simulink model "CurveLowVel"  (R2024b)
settings: Solver=FixedStepAuto  StartTime=0.0  StopTime=Ts  FixedStep=0.001  RelTol=1e-3
PreLoadFcn:
  | setUpCurveLowVel
model workspace (MAT data in the model file):
  firstWarning = 0
  originalScenarioChecksum = 'F73A6DA3C723D3CA73A6F931B7A52A9C'
values from neighbouring files (symbols this model uses):
  K = lqr(A,B,Q,R)    [LQR_Coeff_Low_Vel.m]
  psi_o = 0    [setUpCurveLowVel.m]
  X_o = refPose(1,1)    [setUpCurveLowVel.m]
  xRef = refPose(:,1)    [setUpCurveLowVel.m]
  Y_o = -refPose(1,2)    [setUpCurveLowVel.m]
  yRef = -refPose(:,2)    [setUpCurveLowVel.m]
libraries: simulink x6, slpidlib x2, vehdynlibviscommon x1, autolibshared x1
settings Model: PacingRate=0.700000  Creator=valakshe  LastModifiedBy=Karthik R
settings SolverCC: AlgebraicLoopSolver=TrustRegion
settings OptimizationCC: OptimizeBlockIOStorage=off  OptimizeDataStoreBuffers=off  BusAssignmentInplaceUpdate=off
settings DebuggingCC: UnconnectedInputMsg=warning  UnconnectedOutputMsg=warning  UnconnectedLineMsg=warning  SFUnexpectedBacktrackingDiag=warning  SFNoUnconditionalDefaultTransitionDiag=warning
settings ModelReferenceCC: EnableRefExpFcnMdlSchedulingChecks=on
settings RTWCC: GenerateReport=on  BuildConfiguration=Debug  LaunchReport=on  GPUComputeCapability=3.5  DLArmComputeVersion=19.05
settings CodeAppCC: ForceParamTrailComments=on  MATLABSourceComments=on  EnableCustomComments=on
settings GRTTargetCC: CombineSignalStateStructs=on  SupportVariableSizeSignals=on  MultiInstanceErrorCode=Warning

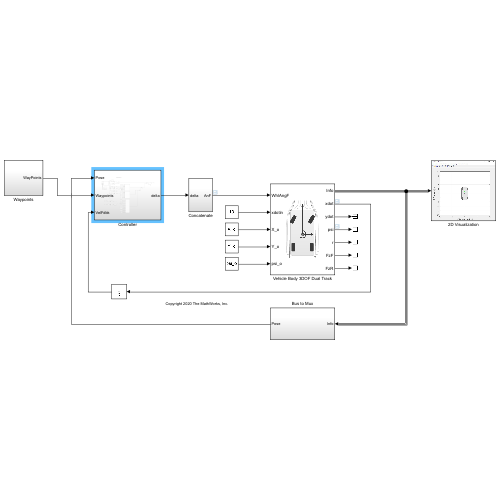
[thumbnail: Simulink's stored preview of the top-level diagram]
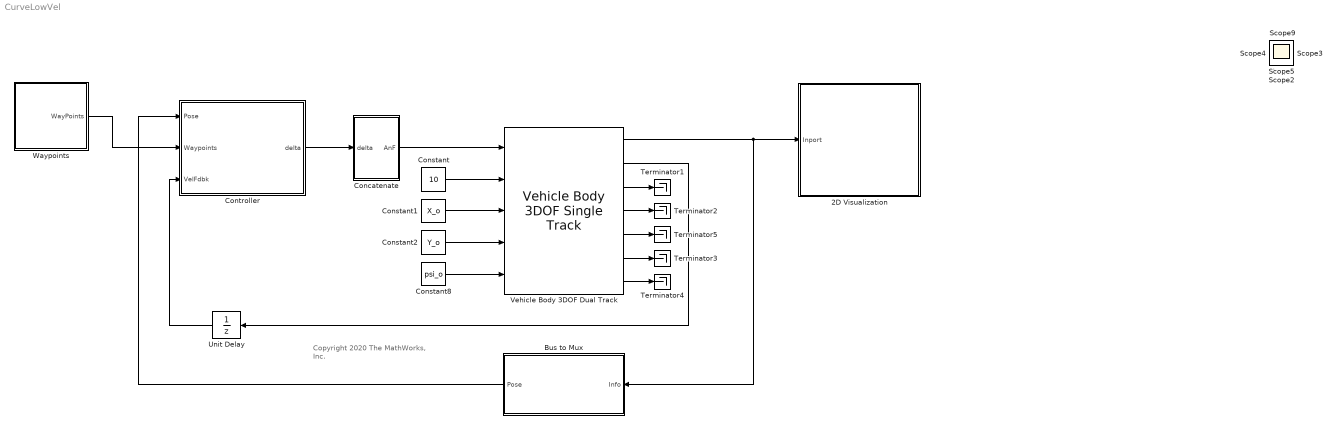
== system CurveLowVel ==
  note: Copyright 2020 The MathWorks, Inc.
  2D Visualization : Subsystem
      mask Display: image("visualization.JPG");
  Bus to Mux : Subsystem
  Concatenate : Subsystem
  Constant : Constant  Value=10
  Constant1 : Constant  Value=X_o
  Constant2 : Constant  Value=Y_o
  Constant8 : Constant  Value=psi_o
  Controller : Subsystem
  Terminator{1..5} (5 alike) : Terminator
  Unit Delay : UnitDelay  SampleTime=-1  HasFrameUpgradeWarning=on
  Vehicle Body 3DOF Dual Track : autolibshared/Vehicle Body 3DOF Single Track  trackMode=Dual  inputMode=External longitudinal velocity  frontSteerMode=on  rearSteerMode=off  windMode=off  muMode=off  extFMode=off  extMMode=off  htchFMode=off  htchMMode=off  extXo=on  extpsio=on  extxdoto=off  extro=off  extYo=on  extTamb=off  extydoto=off  aMode=2  NF=2  NR=2  m=2000  a=1.4  b=1.6  h=0.35  dh=1  hh=0.2  X_o=0  xdot_o=0  CalphaMode=off  sigmaMode=on  d=0  hl=0  w=[1.4,1.4]  Cy_f=12e3  Cy_r=11e3  sigma_f=.1  sigma_r=.1  alpha_f_brk=[-.1 .1]  Cy_f_data=[-9e3 9e3]  alpha_r_brk=[-.1 .1]  Cy_r_data=[-9e3 9e3]  Y_o=0  ydot_o=0  Izz=4000  psi_o=0  r_o=0  Af=2  Cd=.3  Cl=.1  Cpm=.1  beta_w=[0:0.01:0.3]  Cs=[0:0.03:0.9]  Cym=[0:0.01:0.3]  Pabs=101325  Tair=273  g=9.81  mu=1  xdot_tol=.01  Fznom=5000  Fxtire_sat=7e4  Fytire_sat=7e4  longOff=0  latOff=0  vertOff=0  wrapAng=off
  Waypoints : Subsystem
  Scope{,1..5,9} (7 alike) : Scope
  wires:
  Vehicle Body 3DOF Dual Track/7 -> Terminator4/1
  Vehicle Body 3DOF Dual Track/3 -> Terminator1/1
  Constant1/1 -> Vehicle Body 3DOF Dual Track/3
  Vehicle Body 3DOF Dual Track/6 -> Terminator3/1
  Constant2/1 -> Vehicle Body 3DOF Dual Track/4
  Concatenate/1(AnF) -> Vehicle Body 3DOF Dual Track/1
  Constant8/1 -> Vehicle Body 3DOF Dual Track/5
  Vehicle Body 3DOF Dual Track/1 -> 2D Visualization/1(Inport), Bus to Mux/1(Info)
  Controller/1(delta) -> Concatenate/1(delta)
  Bus to Mux/1(Pose) -> Controller/1(Pose)
  Constant/1 -> Vehicle Body 3DOF Dual Track/2
  Vehicle Body 3DOF Dual Track/4 -> Terminator2/1
  Vehicle Body 3DOF Dual Track/5 -> Terminator5/1
  Vehicle Body 3DOF Dual Track/2 -> Unit Delay/1
  Waypoints/1(WayPoints) -> Controller/2(Waypoints)
  Unit Delay/1 -> Controller/3(VelFdbk)

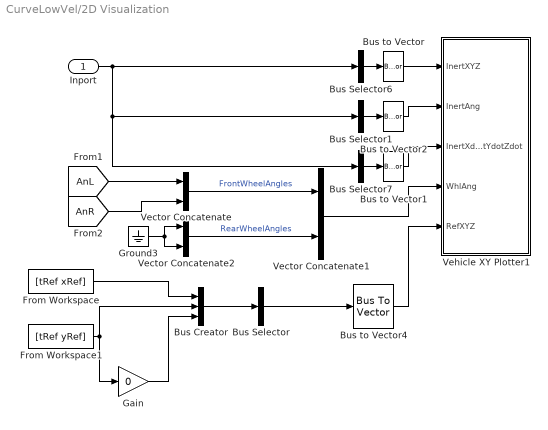
== system CurveLowVel/2D Visualization ==
  Inport : Inport
  Bus Creator : BusCreator  Inputs=3
  Bus Selector : BusSelector  OutputSignals=signal1,signal2,signal3  OutputAsBus=on
  Bus Selector1 : BusSelector  OutputSignals=InertFrm.Cg.Ang.phi,InertFrm.Cg.Ang.theta,InertFrm.Cg.Ang.psi  OutputAsBus=on
  Bus Selector6 : BusSelector  OutputSignals=InertFrm.Geom.Disp.X,InertFrm.Geom.Disp.Y,InertFrm.Geom.Disp.Z  OutputAsBus=on
  Bus Selector7 : BusSelector  OutputSignals=InertFrm.Geom.Vel.Xdot,InertFrm.Geom.Vel.Ydot,InertFrm.Geom.Vel.Zdot  OutputAsBus=on
  Bus to Vector{,1..2,4} (4 alike) : BusToVector
  From Workspace : FromWorkspace  VariableName=[tRef xRef]
  From Workspace1 : FromWorkspace  VariableName=[tRef yRef]
  Gain : Gain  Gain=0
  Ground3 : Ground
  Vector Concatenate : Concatenate
  Vector Concatenate1 : Concatenate
  Vector Concatenate2 : Concatenate
  Vehicle XY Plotter1 : Subsystem  mask(Vehicle XY Plotter){extRef=on, extStats=off, extTireF=off, a=2, b=2, w=2, figBorder=10, bufferSize=1024, velNorm=5, tireFNorm=1000, pltDT=0.2}
      mask prompts: extRef "Plot path reference, extRef"; extStats "Display speed, RPM and Gear"; extTireF "Display tire forces"; a "Distance to front axle from CG, a [m]:"; b "Distance to rear axle from CG, b [m]:"; w "Track width, w [m]:"; figBorder "Distance to figure borders, figBorder [m]:"; bufferSize "Path buffer sampe size, bufferSize []:"; velNorm "Velocity vector scaling, velNorm [m*s/m]:"; tireFNorm "Tire force vector scaling, tireFNorm [m/N]:"; pltDT "Plot update rate, pltDT [s]:"
      mask help:
      | This block will display a MATLAB figure which indicates the vehicle path, current position and heading velocity.
      | An optional path reference is also provided.
      mask init:
      | block = gcb;
      | if autoblkschecksimstopped(block)
      |     ParamNames = {'extRef';'extStats';'extTireF';'extTireF'};
      |     PortNames = {'RefXYZ';'Stats';'TireFx';'TireFy'};
      |     for idx=1:length(PortNames)
      |         InportOption  = {'built-in/Ground', [PortNames{idx}, ' Ground'];...
      |             'built-in/Inport',PortNames{idx}};
      |         if ~strcmp(get_param(block,ParamNames{idx}),'on')
      |             NewBlkHdl = autoblksreplaceblock(block, InportOption, 1);
      |             set_param(NewBlkHdl, 'ShowName', 'off');
      |         else
      |             autoblksreplaceblock(block, InportOption, 2);
      |         end
      |     end
      |     InportNames = {'InertXYZ';'InertAng';'InertXdotYdotZdot';'WhlAng';'RefXYZ';'Stats';'TireFx';'TireFy'};
      |     FoundNames = get_param(find_system(block, 'LookUnderMasks', 'all', 'SearchDepth', 1, 'FollowLinks', 'on', 'BlockType', 'Inport'), 'Name');
      |     [~,PortI] = intersect(InportNames, FoundNames);
      |     PortI = sort(PortI);
      |     for idx = 1:length(PortI)
      |         set_param([block, '/', InportNames{PortI(idx)}], 'Port', num2str(idx));
      |     end
      | end
      mask TypeOptions a: Vehicle XY Plotter/a
      mask TypeOptions b: Vehicle XY Plotter/b
      mask TypeOptions w: Vehicle XY Plotter/w
      mask TypeOptions figBorder: Vehicle XY Plotter/figBorder
      mask TypeOptions bufferSize: Vehicle XY Plotter/bufferSize
      mask TypeOptions velNorm: Vehicle XY Plotter/velNorm
      mask TypeOptions tireFNorm: Vehicle XY Plotter/tireFNorm
      mask DialogControl Container3 Prompt: Plot and Display Options
  wires:
  Vector Concatenate1/1 -> Vehicle XY Plotter1/4(WhlAng)
  Ground3/1 -> Vector Concatenate2/1, Vector Concatenate2/2
  Bus Selector6/1 -> Bus to Vector/1
  Vector Concatenate/1 -> Vector Concatenate1/1  "FrontWheelAngles"
  [AnL] -> Vector Concatenate/1
  Vector Concatenate2/1 -> Vector Concatenate1/2  "RearWheelAngles"
  Bus Selector7/1 -> Bus to Vector1/1
  Bus to Vector1/1 -> Vehicle XY Plotter1/3(InertXdotYdotZdot)
  Bus to Vector/1 -> Vehicle XY Plotter1/1(InertXYZ)
  Bus to Vector2/1 -> Vehicle XY Plotter1/2(InertAng)
  Bus Selector1/1 -> Bus to Vector2/1
  [AnR] -> Vector Concatenate/2
  Inport/1 -> Bus Selector7/1, Bus Selector1/1, Bus Selector6/1
  Bus to Vector4/1 -> Vehicle XY Plotter1/5(RefXYZ)
  Bus Selector/1 -> Bus to Vector4/1
  From Workspace1/1 -> Gain/1, Bus Creator/2
  Gain/1 -> Bus Creator/3
  From Workspace/1 -> Bus Creator/1
  Bus Creator/1 -> Bus Selector/1

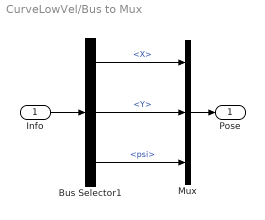
== system CurveLowVel/Bus to Mux ==
  Info : Inport
  Bus Selector1 : BusSelector  OutputSignals=InertFrm.Cg.Disp.X,InertFrm.Cg.Disp.Y,InertFrm.Cg.Ang.psi
  Mux : Mux  Inputs=3
  Pose : Outport
  wires:
  Bus Selector1/3 -> Mux/3  "<psi>"
  Bus Selector1/1 -> Mux/1  "<X>"
  Mux/1 -> Pose/1
  Bus Selector1/2 -> Mux/2  "<Y>"
  Info/1 -> Bus Selector1/1

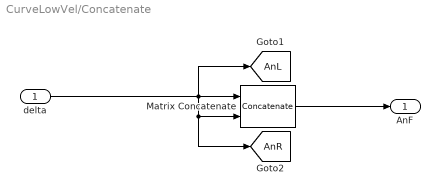
== system CurveLowVel/Concatenate ==
  delta : Inport
  Matrix Concatenate : Concatenate
  AnF : Outport  VectorParamsAs1DForOutWhenUnconnected=off
  tag scope: AnL=global, AnR=global
  wires:
  Matrix Concatenate/1 -> AnF/1
  delta/1 -> [AnL], [AnR], Matrix Concatenate/2, Matrix Concatenate/1

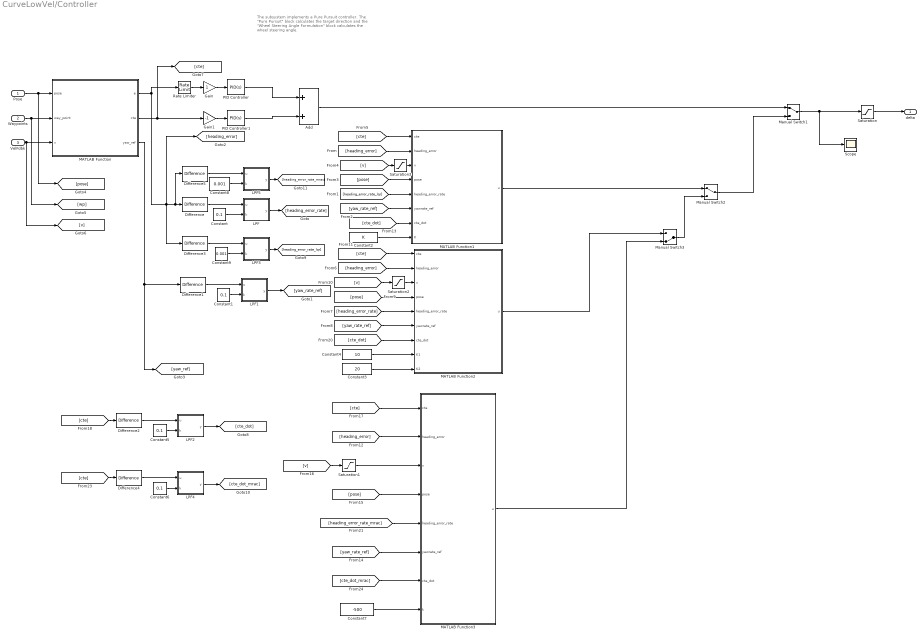
== system CurveLowVel/Controller ==
  note: The subsystem implements a Pure Pursuit controller. The "Pure Pursuit" block calculates the target direction and the "Wheel Steering Angle Formulation" block calculates the wheel steering angle.
  Pose : Inport
  Waypoints : Inport  Port=2
  VelFdbk : Inport  Port=3
  Add : Sum
  Constant{,1,5..6} (4 alike) : Constant  Value=0.1
  Constant2 : Constant  Value=K
  Constant3 : Constant  Value=20
  Constant4 : Constant  Value=10
  Constant7 : Constant  Value=-500
  Constant8 : Constant  Value=0.001
  Constant9 : Constant  Value=0.001
  Difference{,1..5} (6 alike) : simulink/Discrete/Difference  ICPrevInput=0.0  OutMin=[]  OutMax=[]  OutDataType=fixdt(1, 16)  OutScaling=2^-10  DoSatur=off
  Gain : Gain
  Gain1 : Gain  Gain=-1
  LPF : Subsystem
  LPF1 : Subsystem
  LPF2 : Subsystem
  LPF3 : Subsystem
  LPF4 : Subsystem
  LPF5 : Subsystem
  MATLAB Function : MATLAB Function  TreatAsAtomicUnit=on
  MATLAB Function1 : MATLAB Function  TreatAsAtomicUnit=on
  MATLAB Function2 : MATLAB Function  TreatAsAtomicUnit=on
  MATLAB Function3 : MATLAB Function  TreatAsAtomicUnit=on
  Manual Switch1 : ManualSwitch
  Manual Switch2 : ManualSwitch
  Manual Switch3 : ManualSwitch  CurrentSetting=0
  PID Controller : slpidlib/PID Controller  Controller=PID  Form=Parallel  TimeDomain=Continuous-time  UseExternalTs=off  SampleTime=-1  IntegratorMethod=Forward Euler  FilterMethod=Forward Euler  ControllerParametersSource=internal  P=0.7  I=0.002  UseKiTs=off  D=0  UseExternalDerivativeSource=off  N=100  UseFilter=on  TunerSelectOption=Transfer Function Based (PID Tuner App)  InitialConditionSource=internal  InitialConditionForIntegrator=0  InitialConditionForFilter=0  DifferentiatorICPrevScaledInput=0  ExternalReset=none  TrackingMode=off  Kt=1  LimitOutput=off  SatLimitsSource=internal  UpperSaturationLimit=inf  LowerSaturationLimit=-inf  LinearizeAsGain=on  AntiWindupMode=none  Kb=1  LimitIntegrator=off  UpperIntegratorSaturationLimit=inf  LowerIntegratorSaturationLimit=-inf  POutMin=[]  POutMax=[]  IOutMin=[]  IOutMax=[]  DOutMin=[]  DOutMax=[]  NOutMin=[]  NOutMax=[]  SumOutMin=[]  SumOutMax=[]  SaturationOutMin=[]  SaturationOutMax=[]  PParamMin=[]  PParamMax=[]  IParamMin=[]  IParamMax=[]  DParamMin=[]  DParamMax=[]  NParamMin=[]  NParamMax=[]  KbParamMin=[]  KbParamMax=[]  KtParamMin=[]  KtParamMax=[]  KbOutMin=[]  KbOutMax=[]  KtOutMin=[]  KtOutMax=[]  IntegratorOutMin=[]  IntegratorOutMax=[]  FilterOutMin=[]  FilterOutMax=[]  SumI1OutMin=[]  SumI1OutMax=[]  SumI2OutMin=[]  SumI2OutMax=[]  SumI3OutMin=[]  SumI3OutMax=[]  SumI4OutMin=[]  SumI4OutMax=[]  SumDOutMin=[]  SumDOutMax=[]  DifferentiatorOutMin=[]  DifferentiatorOutMax=[]  FilterDiffOutCoefMin=[]  FilterDiffOutCoefMax=[]  ReciprocalOutMin=[]  ReciprocalOutMax=[]  SumDenOutMin=[]  SumDenOutMax=[]  SumNumOutMin=[]  SumNumOutMax=[]  DivideOutMin=[]  DivideOutMax=[]  UdiffTsProdOutMin=[]  UdiffTsProdOutMax=[]  NTsProdOutMin=[]  NTsProdOutMax=[]  UintegralTsProdOutMin=[]  UintegralTsProdOutMax=[]  UngainTsProdOutMin=[]  UngainTsProdOutMax=[]  ClampingZeroOutDataTypeStr=Inherit: Inherit via back propagation  ClampingZeroOutMin=[]  ClampingZeroOutMax=[]  FilterDenConstantOutDataTypeStr=Inherit: Inherit via back propagation  FilterDenConstantOutMin=[]  FilterDenConstantOutMax=[]  PCopyOutDataTypeStr=Inherit: Inherit via back propagation  PCopyOutMin=[]  PCopyOutMax=[]  NCopyOutDataTypeStr=Inherit: Inherit via back propagation  NCopyOutMin=[]  NCopyOutMax=[]  IntegratorContinuousStateAttributes=''  IntegratorStateMustResolveToSignalObject=off  IntegratorRTWStateStorageClass=Auto  FilterContinuousStateAttributes=''  FilterStateMustResolveToSignalObject=off  FilterRTWStateStorageClass=Auto  ParallelPVariant=InternalParameters  IdealPVariant=Disabled  IVariant=InternalParameters  DVariant=InternalParameters  IntegratorVariant=Continuous  SatVariant=Disabled  AWVariant=Passthrough  PCopyVariant=Disabled  TRVariant=Disabled  FdbkBlocksVariant=Forward  IdealPFdbkVariant=Disabled  SatFdbkVariant=Disabled  DerivativeFilterVariant=ContFilter  NVariant=InternalParameters  NCopyVariant=Disabled  FilterICVariant=InternalICsFilter  IntegratorICVariant=InternalICs  ExternalResetVariant=Disabled  TRSumVariant=Passthrough  SumFdbkVariant=Disabled  SumVariant=Sum_PID  TsampFilterVariant=InternalTs  TsampNgainVariant=Passthrough  TsampIntegralVariant=Disabled_SignalSpec  ExternalSaturationOutDataTypeStr=Inherit: Same as second input  DerivativeSourceVariant=ErrorSignal  PreIntVariant=InternalPreInt
  PID Controller1 : slpidlib/PID Controller  Controller=PID  Form=Parallel  TimeDomain=Continuous-time  UseExternalTs=off  SampleTime=-1  IntegratorMethod=Forward Euler  FilterMethod=Forward Euler  ControllerParametersSource=internal  P=0.07  I=0.0002  UseKiTs=off  D=0  UseExternalDerivativeSource=off  N=100  UseFilter=on  TunerSelectOption=Transfer Function Based (PID Tuner App)  InitialConditionSource=internal  InitialConditionForIntegrator=0  InitialConditionForFilter=0  DifferentiatorICPrevScaledInput=0  ExternalReset=none  TrackingMode=off  Kt=1  LimitOutput=off  SatLimitsSource=internal  UpperSaturationLimit=inf  LowerSaturationLimit=-inf  LinearizeAsGain=on  AntiWindupMode=none  Kb=1  LimitIntegrator=off  UpperIntegratorSaturationLimit=inf  LowerIntegratorSaturationLimit=-inf  POutMin=[]  POutMax=[]  IOutMin=[]  IOutMax=[]  DOutMin=[]  DOutMax=[]  NOutMin=[]  NOutMax=[]  SumOutMin=[]  SumOutMax=[]  SaturationOutMin=[]  SaturationOutMax=[]  PParamMin=[]  PParamMax=[]  IParamMin=[]  IParamMax=[]  DParamMin=[]  DParamMax=[]  NParamMin=[]  NParamMax=[]  KbParamMin=[]  KbParamMax=[]  KtParamMin=[]  KtParamMax=[]  KbOutMin=[]  KbOutMax=[]  KtOutMin=[]  KtOutMax=[]  IntegratorOutMin=[]  IntegratorOutMax=[]  FilterOutMin=[]  FilterOutMax=[]  SumI1OutMin=[]  SumI1OutMax=[]  SumI2OutMin=[]  SumI2OutMax=[]  SumI3OutMin=[]  SumI3OutMax=[]  SumI4OutMin=[]  SumI4OutMax=[]  SumDOutMin=[]  SumDOutMax=[]  DifferentiatorOutMin=[]  DifferentiatorOutMax=[]  FilterDiffOutCoefMin=[]  FilterDiffOutCoefMax=[]  ReciprocalOutMin=[]  ReciprocalOutMax=[]  SumDenOutMin=[]  SumDenOutMax=[]  SumNumOutMin=[]  SumNumOutMax=[]  DivideOutMin=[]  DivideOutMax=[]  UdiffTsProdOutMin=[]  UdiffTsProdOutMax=[]  NTsProdOutMin=[]  NTsProdOutMax=[]  UintegralTsProdOutMin=[]  UintegralTsProdOutMax=[]  UngainTsProdOutMin=[]  UngainTsProdOutMax=[]  ClampingZeroOutDataTypeStr=Inherit: Inherit via back propagation  ClampingZeroOutMin=[]  ClampingZeroOutMax=[]  FilterDenConstantOutDataTypeStr=Inherit: Inherit via back propagation  FilterDenConstantOutMin=[]  FilterDenConstantOutMax=[]  PCopyOutDataTypeStr=Inherit: Inherit via back propagation  PCopyOutMin=[]  PCopyOutMax=[]  NCopyOutDataTypeStr=Inherit: Inherit via back propagation  NCopyOutMin=[]  NCopyOutMax=[]  IntegratorContinuousStateAttributes=''  IntegratorStateMustResolveToSignalObject=off  IntegratorRTWStateStorageClass=Auto  FilterContinuousStateAttributes=''  FilterStateMustResolveToSignalObject=off  FilterRTWStateStorageClass=Auto  ParallelPVariant=InternalParameters  IdealPVariant=Disabled  IVariant=InternalParameters  DVariant=InternalParameters  IntegratorVariant=Continuous  SatVariant=Disabled  AWVariant=Passthrough  PCopyVariant=Disabled  TRVariant=Disabled  FdbkBlocksVariant=Forward  IdealPFdbkVariant=Disabled  SatFdbkVariant=Disabled  DerivativeFilterVariant=ContFilter  NVariant=InternalParameters  NCopyVariant=Disabled  FilterICVariant=InternalICsFilter  IntegratorICVariant=InternalICs  ExternalResetVariant=Disabled  TRSumVariant=Passthrough  SumFdbkVariant=Disabled  SumVariant=Sum_PID  TsampFilterVariant=InternalTs  TsampNgainVariant=Passthrough  TsampIntegralVariant=Disabled_SignalSpec  ExternalSaturationOutDataTypeStr=Inherit: Same as second input  DerivativeSourceVariant=ErrorSignal  PreIntVariant=InternalPreInt
  Rate Limiter : RateLimiter  RisingSlewLimit=10  FallingSlewLimit=-10  SampleTimeMode=inherited
  Saturation : Saturate  UpperLimit=3  LowerLimit=-3
  Saturation1 : Saturate  UpperLimit=200  LowerLimit=1
  Saturation2 : Saturate  UpperLimit=200  LowerLimit=1
  Saturation3 : Saturate  UpperLimit=200  LowerLimit=3
  Scope : Scope
  delta : Outport
  wires:
  Waypoints/1 -> [wp], MATLAB Function/2(way_point)
  Pose/1 -> [pose], MATLAB Function/1(pose)
  Manual Switch1/1 -> Scope/1, Saturation/1
  VelFdbk/1 -> [v], MATLAB Function/3(v)
  Rate Limiter/1 -> Gain/1
  Gain/1 -> PID Controller/1
  Add/1 -> Manual Switch1/1
  PID Controller/1 -> Add/1
  PID Controller1/1 -> Add/2
  MATLAB Function/2(cte) -> [cte], Gain1/1
  Gain1/1 -> PID Controller1/1
  Difference/1 -> LPF/1(u)
  MATLAB Function/3(yaw_ref) -> [yaw_ref], Difference1/1
  Difference1/1 -> LPF1/1(u)
  Constant/1 -> LPF/2(k)
  Constant1/1 -> LPF1/2(k)
  Constant2/1 -> MATLAB Function1/8(K)
  MATLAB Function1/1(u) -> Manual Switch2/1
  Manual Switch2/1 -> Manual Switch1/2
  MATLAB Function2/1(u) -> Manual Switch3/1
  Constant3/1 -> MATLAB Function2/9(K2)
  Constant4/1 -> MATLAB Function2/8(K1)
  Saturation/1 -> delta/1
  MATLAB Function3/1(u) -> Manual Switch3/2
  Manual Switch3/1 -> Manual Switch2/2
  LPF/1(y) -> [heading_error_rate]
  LPF1/1(y) -> [yaw_rate_ref]
  [heading_error] -> MATLAB Function1/2(heading_error)
  [heading_error_rate_lqr] -> MATLAB Function1/5(heading_error_rate)
  [yaw_rate_ref] -> MATLAB Function1/6(yawrate_ref)
  [pose] -> MATLAB Function1/4(pose)
  [v] -> Saturation3/1
  [cte] -> MATLAB Function1/1(cte)
  [cte] -> MATLAB Function2/1(cte)
  [heading_error] -> MATLAB Function2/2(heading_error)
  [v] -> Saturation2/1
  [pose] -> MATLAB Function2/4(pose)
  [heading_error_rate] -> MATLAB Function2/5(heading_error_rate)
  [yaw_rate_ref] -> MATLAB Function2/6(yawrate_ref)
  [cte] -> MATLAB Function3/1(cte)
  [heading_error] -> MATLAB Function3/2(heading_error)
  [v] -> Saturation1/1
  [pose] -> MATLAB Function3/4(pose)
  [heading_error_rate_mrac] -> MATLAB Function3/5(heading_error_rate)
  [yaw_rate_ref] -> MATLAB Function3/6(yawrate_ref)
  LPF2/1(y) -> [cte_dot]
  [cte] -> Difference2/1
  Constant5/1 -> LPF2/2(k)
  Difference2/1 -> LPF2/1(u)
  [cte_dot_mrac] -> MATLAB Function3/7(cte_dot)
  Saturation1/1 -> MATLAB Function3/3(v)
  Saturation2/1 -> MATLAB Function2/3(v)
  Saturation3/1 -> MATLAB Function1/3(v)
  [cte_dot] -> MATLAB Function2/7(cte_dot)
  Constant7/1 -> MATLAB Function3/8(k)
  LPF3/1(y) -> [heading_error_rate_lqr]
  Difference3/1 -> LPF3/1(u)
  Constant9/1 -> LPF3/2(k)
  [cte_dot] -> MATLAB Function1/7(cte_dot)
  Difference4/1 -> LPF4/1(u)
  [cte] -> Difference4/1
  Constant6/1 -> LPF4/2(k)
  LPF4/1(y) -> [cte_dot_mrac]
  MATLAB Function/1(e) -> Difference3/1, [heading_error], Difference5/1, Difference/1, Rate Limiter/1
  LPF5/1(y) -> [heading_error_rate_mrac]
  Constant8/1 -> LPF5/2(k)
  Difference5/1 -> LPF5/1(u)

== system CurveLowVel/Waypoints ==
  Constant3 : Constant  Value=xRef  SampleTime=0.1
  Constant4 : Constant  Value=yRef  SampleTime=0.1
  Matrix Concatenate : Concatenate  Mode=Multidimensional array  ConcatenateDimension=2
  WayPoints : Outport
  wires:
  Constant4/1 -> Matrix Concatenate/2
  Constant3/1 -> Matrix Concatenate/1
  Matrix Concatenate/1 -> WayPoints/1

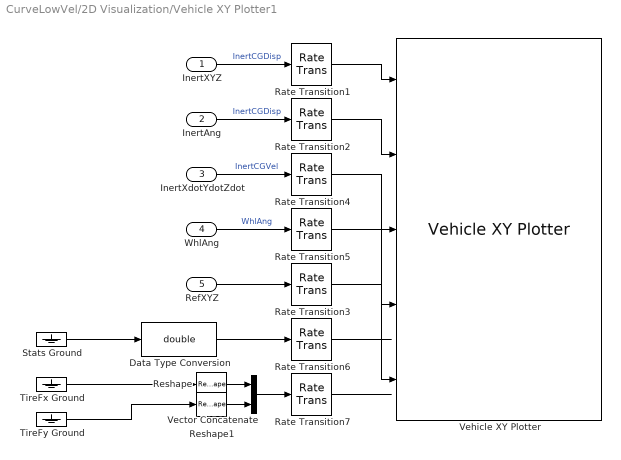
== system CurveLowVel/2D Visualization/Vehicle XY Plotter1 ==
  InertXYZ : Inport
  InertAng : Inport  Port=2
  InertXdotYdotZdot : Inport  Port=3
  WhlAng : Inport  Port=4
  RefXYZ : Inport  Port=5
  Data Type Conversion : DataTypeConversion  OutDataTypeStr=double  SaturateOnIntegerOverflow=off  RndMeth=Floor
  Rate Transition{1..7} (7 alike) : RateTransition  Deterministic=off  OutPortSampleTime=pltDT
  Reshape : Reshape  OutputDimensionality=Row vector (2-D)
  Reshape1 : Reshape  OutputDimensionality=Row vector (2-D)
  Stats Ground : Ground
  TireFx Ground : Ground
  TireFy Ground : Ground
  Vector Concatenate : Concatenate  Mode=Multidimensional array
  Vehicle XY Plotter : vehdynlibviscommon/Vehicle XY Plotter  w=w  a=a  b=b  figBorder=figBorder  bufferSize=bufferSize  extStats=off  extTireF=off
  wires:
  Vector Concatenate/1 -> Rate Transition7/1
  Reshape1/1 -> Vector Concatenate/2
  Reshape/1 -> Vector Concatenate/1
  RefXYZ/1 -> Rate Transition3/1
  Rate Transition7/1 -> ?
  Data Type Conversion/1 -> Rate Transition6/1
  Rate Transition6/1 -> ?
  Rate Transition5/1 -> Vehicle XY Plotter/4
  Rate Transition4/1 -> Vehicle XY Plotter/3
  Rate Transition2/1 -> Vehicle XY Plotter/2
  Rate Transition1/1 -> Vehicle XY Plotter/1
  Rate Transition3/1 -> Vehicle XY Plotter/5
  WhlAng/1 -> Rate Transition5/1  "WhlAng"
  InertXYZ/1 -> Rate Transition1/1  "InertCGDisp"
  InertXdotYdotZdot/1 -> Rate Transition4/1  "InertCGVel"
  InertAng/1 -> Rate Transition2/1  "InertCGDisp"
  Stats Ground/1 -> Data Type Conversion/1
  TireFx Ground/1 -> Reshape/1
  TireFy Ground/1 -> Reshape1/1

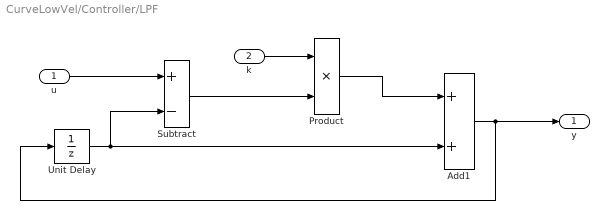
== system CurveLowVel/Controller/LPF ==
  u : Inport
  k : Inport  Port=2
  Add1 : Sum
  Product : Product
  Subtract : Sum  Inputs=+-
  Unit Delay : UnitDelay  SampleTime=-1  HasFrameUpgradeWarning=on
  y : Outport
  wires:
  k/1 -> Product/1
  Product/1 -> Add1/1
  Add1/1 -> y/1, Unit Delay/1
  Unit Delay/1 -> Subtract/2, Add1/2
  u/1 -> Subtract/1
  Subtract/1 -> Product/2

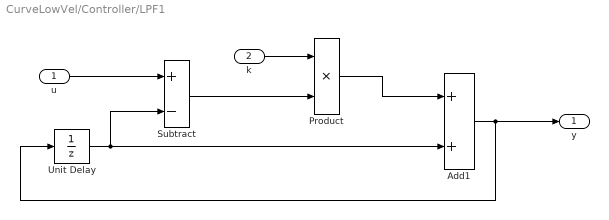
== system CurveLowVel/Controller/LPF1 ==
  u : Inport
  k : Inport  Port=2
  Add1 : Sum
  Product : Product
  Subtract : Sum  Inputs=+-
  Unit Delay : UnitDelay  SampleTime=-1  HasFrameUpgradeWarning=on
  y : Outport
  wires:
  k/1 -> Product/1
  Product/1 -> Add1/1
  Add1/1 -> y/1, Unit Delay/1
  Unit Delay/1 -> Subtract/2, Add1/2
  u/1 -> Subtract/1
  Subtract/1 -> Product/2

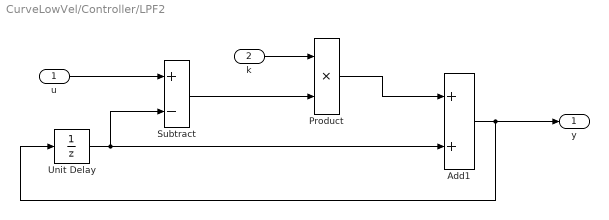
== system CurveLowVel/Controller/LPF2 ==
  u : Inport
  k : Inport  Port=2
  Add1 : Sum
  Product : Product
  Subtract : Sum  Inputs=+-
  Unit Delay : UnitDelay  SampleTime=-1  HasFrameUpgradeWarning=on
  y : Outport
  wires:
  k/1 -> Product/1
  Product/1 -> Add1/1
  Add1/1 -> y/1, Unit Delay/1
  Unit Delay/1 -> Subtract/2, Add1/2
  u/1 -> Subtract/1
  Subtract/1 -> Product/2

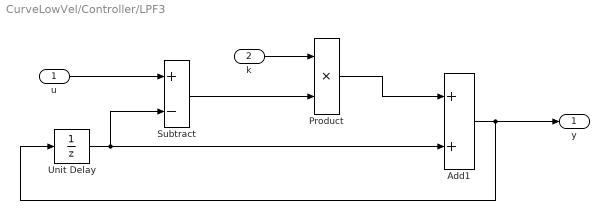
== system CurveLowVel/Controller/LPF3 ==
  u : Inport
  k : Inport  Port=2
  Add1 : Sum
  Product : Product
  Subtract : Sum  Inputs=+-
  Unit Delay : UnitDelay  SampleTime=-1  HasFrameUpgradeWarning=on
  y : Outport
  wires:
  k/1 -> Product/1
  Product/1 -> Add1/1
  Add1/1 -> y/1, Unit Delay/1
  Unit Delay/1 -> Subtract/2, Add1/2
  u/1 -> Subtract/1
  Subtract/1 -> Product/2

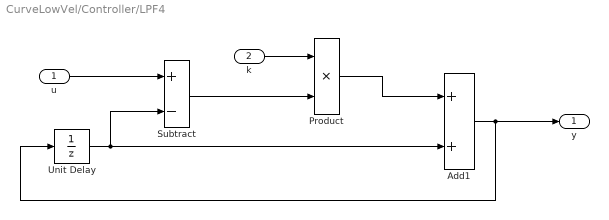
== system CurveLowVel/Controller/LPF4 ==
  u : Inport
  k : Inport  Port=2
  Add1 : Sum
  Product : Product
  Subtract : Sum  Inputs=+-
  Unit Delay : UnitDelay  SampleTime=-1  HasFrameUpgradeWarning=on
  y : Outport
  wires:
  k/1 -> Product/1
  Product/1 -> Add1/1
  Add1/1 -> y/1, Unit Delay/1
  Unit Delay/1 -> Subtract/2, Add1/2
  u/1 -> Subtract/1
  Subtract/1 -> Product/2

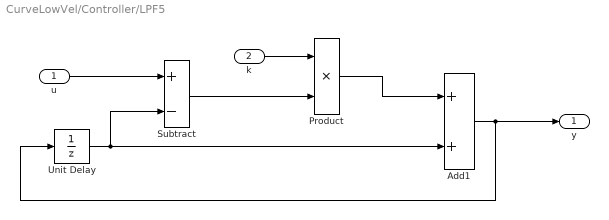
== system CurveLowVel/Controller/LPF5 ==
  u : Inport
  k : Inport  Port=2
  Add1 : Sum
  Product : Product
  Subtract : Sum  Inputs=+-
  Unit Delay : UnitDelay  SampleTime=-1  HasFrameUpgradeWarning=on
  y : Outport
  wires:
  k/1 -> Product/1
  Product/1 -> Add1/1
  Add1/1 -> y/1, Unit Delay/1
  Unit Delay/1 -> Subtract/2, Add1/2
  u/1 -> Subtract/1
  Subtract/1 -> Product/2

== matlab function CurveLowVel/Controller/MATLAB Function ==
  data: pose input; e output; way_point input; v input; cte output; yaw_ref output
function [e,cte,yaw_ref]= error(pose,way_point,v)

    x = pose(1);
    y = pose(2);
    yaw = pose(3);

    nearest_idx = find_nearest_waypoint(x,y,way_point);
    [cte,heading_error,yaw_ref]= compute_cte(x,y,yaw,way_point,nearest_idx,v);    



e = heading_error;
end


function idx = find_nearest_waypoint(x, y, waypoints)
    dists = vecnorm((waypoints - [x, y]).');
    [~, idx] = min(dists);
end
 
function [cte,heading_error,yaw_ref] = compute_cte(x,y,yaw,way_point,idx,v)
    wp1 = way_point(idx,:);
    wp1 = wp1';

    if idx < size(way_point,1)
        wp2 = way_point(idx+1,:);
    else
        wp2 = wp1;
    end
    wp2 = wp2';


    dx = wp2(1) - wp1(1);
    dy = wp2(2) - wp1(2);

    target_angle = atan2(dy, dx);
    heading_error = target_angle - yaw;
    % if heading_error > pi
    %     heading_error = heading_error - 2 * pi;
    % elseif heading_error < -pi
    %     heading_error = heading_error + 2 * pi;
    % end
     

    cte = -sin(yaw) * dx + cos(yaw) * dy;
    cte = v*sin(yaw + heading_error);

    

    seg_vec = [dx,dy];
    pos_vec = [x-wp1(1),y-wp1(2)];
    cross_val = dx * pos_vec(2) - dy * pos_vec(1);
    seg_len = norm(seg_vec) + 1e-6;
    cte = (cross_val / seg_len);
    heading_error = rem(heading_error+pi,2*pi) - pi;
    yaw_ref = target_angle;


    
end

== matlab function CurveLowVel/Controller/MATLAB Function1 ==
  data: cte input; heading_error input; v input; pose input; u output; heading_error_rate input; yawrate_ref input; cte_dot input; K input
function u = lqr(cte,heading_error,v,pose,heading_error_rate,yawrate_ref,cte_dot,K)

    x = pose(1);
    y = pose(2);
    yaw = pose(3);
    Iz = 4000; %kg*m^2
    la = 1.4; %m
    lb = 1.6; %4
    h = 0.35; %m
    m = 2000; %m
    tw = 1.4; %m
    Cf = 2*12000; % N/rad
    Cr = 2*11000; %N/rad
    v = 10;

    
    % cte_dot = v*cos(yaw)*heading_error + v*sin(yaw);
    e_vec = [cte,cte_dot,heading_error,heading_error_rate]';
    
    u = (K(1)*e_vec(1)+K(2)*e_vec(2)+K(3)*e_vec(3)+K(4)*e_vec(4))+heading_error+0.001*yawrate_ref*(la+lb)/10;

 


    

end

== matlab function CurveLowVel/Controller/MATLAB Function2 ==
  data: cte input; heading_error input; v input; pose input; u output; heading_error_rate input; yawrate_ref input; cte_dot input; K1 input; K2 input
function u = smc(cte,heading_error,v,pose,heading_error_rate,yawrate_ref,cte_dot,K1,K2)

    x = pose(1);
    y = pose(2);
    yaw = pose(3);
    Iz = 4000; %kg*m^2
    la = 1.4; %m
    lb = 1.6; %4
    h = 0.35; %m
    m = 2000; %m
    tw = 1.4; %m
    Cf = 2*12000; % N/rad
    Cr = 2*11000; %N/rad
    v = 10;
    temp2 = -(Cf + Cr)/m;
    temp1 = -(Cf*la - Cr*lb);
    temp3 = -(Cf*la^2 + Cr*lb^2)/v/Iz;



    
    % cte_dot = v*cos(yaw)*heading_error + v*sin(yaw);
    e_vec = [cte,cte_dot,heading_error,heading_error_rate]';

    c1 = 0.07;
    c2 = 0.0005;

    s = c1*cte_dot + c2*heading_error;
    
    u = -m*(-(temp1/m/v - v)*yawrate_ref - temp2*cte_dot/v + temp2*heading_error - temp2*(heading_error_rate)/m/v - K1 *tanh(s) - c2*heading_error_rate/c1 - K2*s )/Cf;

    

end

== matlab function CurveLowVel/Controller/MATLAB Function3 ==
  data: cte input; heading_error input; v input; pose input; u output; heading_error_rate input; yawrate_ref input; cte_dot input; k input
function u  = mrac(cte,heading_error,v,pose,heading_error_rate,yawrate_ref,cte_dot,k)


    x = pose(1);
    y = pose(2);
    yaw = pose(3);
    
    Iz = 4000; %kg*m^2
    la = 1.4; %m
    lb = 1.6; %4
    h = 0.35; %m
    m = 2000; %m
    tw = 1.4; %m
    Cf = 2*12000; % N/rad
    Cr = 2*11000; %N/rad

    % 


    % cte_dot = v*cos(yaw)*heading_error + v*sin(yaw);
        c2 = (Cf*la - Cr*lb)/Iz;
        c1 = -c2/v;
        c3 = -(Cf*la^2 + Cr*lb^2)/Iz/v;
    
       u = -(k*heading_error_rate + c1*cte_dot + c2*heading_error + c3*heading_error_rate + c3*yawrate_ref);









end
